simulink model "Boost_model_closed"  (R2021a)
settings: Solver=VariableStepAuto  StartTime=0.0  StopTime=100*1e-3  FixedStep=1e-6  MaxStep=1e-7  RelTol=1e-3
undefined symbols (not defined in the file): bits, DCR, ESR_Cout, f_s, general, gmis_v, K_i_0, K_p_0, nlsb_v, ofs_v, sat_v, T_A2D, t_f, T_PWM, tf1, V_out, V_out_p
libraries: fl_lib x14, ee_lib x8, nesl_utility x6, spsPWMGeneratorDCDCLib x2
settings Model: Creator=delta  LastModifiedBy=delta
settings SolverCC: MaxConsecutiveMinStep=10  ZeroCrossAlgorithm=Adaptive
settings DebuggingCC: IgnoredZcDiagnostic=none  ParameterOverflowMsg=warning

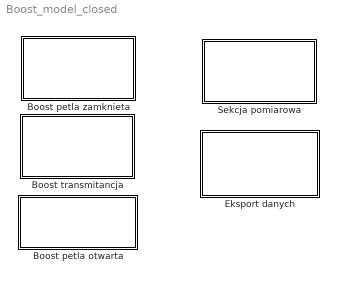
== system Boost_model_closed ==
  Boost petla otwarta : Subsystem
  Boost petla zamknieta : Subsystem
  Boost transmitancja : Subsystem
  Eksport danych : Subsystem
  Sekcja pomiarowa : Subsystem

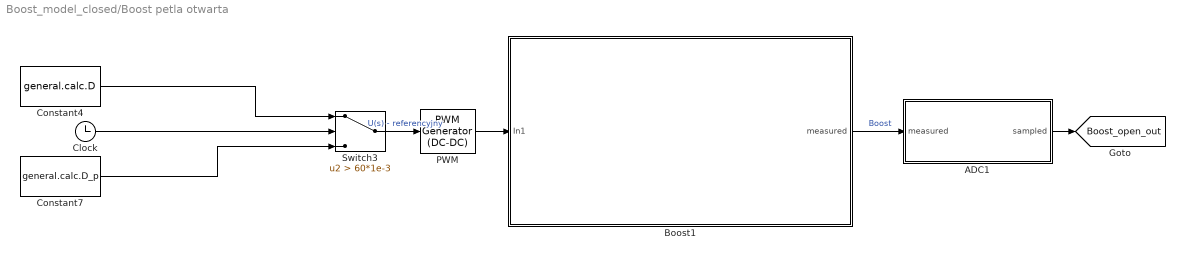
== system Boost_model_closed/Boost petla otwarta ==
  ADC1 : Subsystem
  Boost1 : Subsystem
  Clock : Clock
  Constant4 : Constant  Value=general.calc.D
  Constant7 : Constant  Value=general.calc.D_p
  "PWM " : spsPWMGeneratorDCDCLib/PWM Generator (DC-DC)  Fsw=1/T_PWM  Ts=0
  Switch3 : Switch  Criteria=u2 > Threshold  Threshold=60*1e-3
  tag scope: Boost_open_out=global
  wires:
  ADC1/1(sampled) -> [Boost_open_out]
  Switch3/1 -> "PWM "/1  "U(s) - referencyjny"
  "PWM "/1 -> Boost1/1(In1)
  Clock/1 -> Switch3/2
  Constant4/1 -> Switch3/1
  Boost1/1(measured) -> ADC1/1(measured)  "Boost"
  Constant7/1 -> Switch3/3

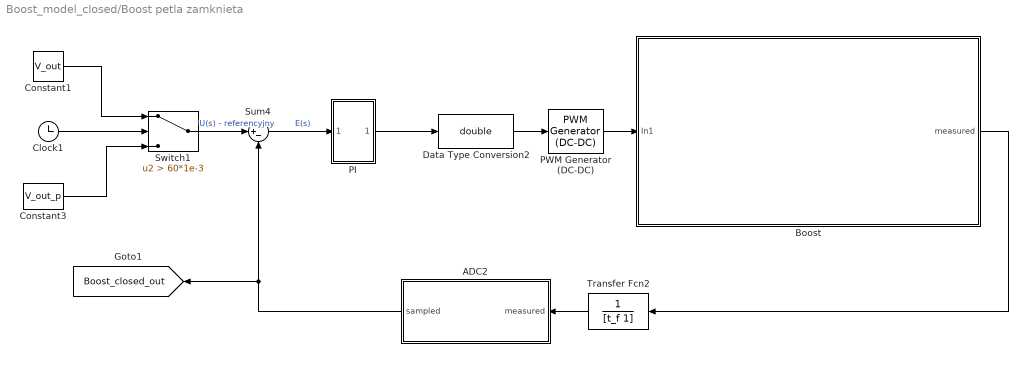
== system Boost_model_closed/Boost petla zamknieta ==
  ADC2 : Subsystem
  Boost : Subsystem
  Clock1 : Clock
  Constant1 : Constant  Value=V_out
  Constant3 : Constant  Value=V_out_p
  Data Type Conversion2 : DataTypeConversion  OutDataTypeStr=double
  PI : Subsystem
  PWM Generator (DC-DC) : spsPWMGeneratorDCDCLib/PWM Generator (DC-DC)  Fsw=1/T_PWM  Ts=0
  Sum4 : Sum  Inputs=|+-
  Switch1 : Switch  Criteria=u2 > Threshold  Threshold=60*1e-3
  Transfer Fcn2 : TransferFcn  Numerator=1  Denominator=[t_f 1]
  tag scope: Boost_closed_out=global
  wires:
  PI/1(Out1) -> Data Type Conversion2/1
  Sum4/1 -> PI/1(In1)  "E(s)"
  Boost/1(measured) -> Transfer Fcn2/1
  Constant3/1 -> Switch1/3
  Clock1/1 -> Switch1/2
  Constant1/1 -> Switch1/1
  ADC2/1(sampled) -> [Boost_closed_out], Sum4/2
  PWM Generator (DC-DC)/1 -> Boost/1(In1)
  Switch1/1 -> Sum4/1  "U(s) - referencyjny"
  Data Type Conversion2/1 -> PWM Generator (DC-DC)/1
  Transfer Fcn2/1 -> ADC2/1(measured)

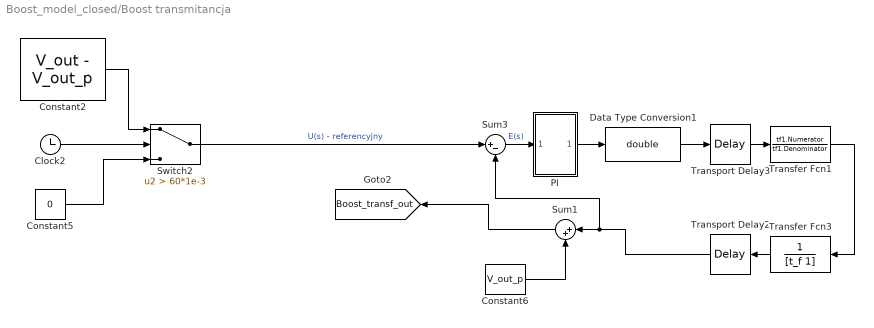
== system Boost_model_closed/Boost transmitancja ==
  Clock2 : Clock
  Constant2 : Constant  Value=V_out - V_out_p
  Constant5 : Constant  Value=0
  Constant6 : Constant  Value=V_out_p
  Data Type Conversion1 : DataTypeConversion  OutDataTypeStr=double
  PI : Subsystem
  Sum1 : Sum  Inputs=|++
  Sum3 : Sum  Inputs=|+-
  Switch2 : Switch  Criteria=u2 > Threshold  Threshold=60*1e-3
  Transfer Fcn1 : TransferFcn  Numerator=tf1.Numerator  Denominator=tf1.Denominator
  Transfer Fcn3 : TransferFcn  Numerator=1  Denominator=[t_f 1]
  Transport Delay2 : TransportDelay  DelayTime=T_A2D
  Transport Delay3 : TransportDelay  DelayTime=T_PWM
  tag scope: Boost_transf_out=global
  wires:
  Transport Delay3/1 -> Transfer Fcn1/1
  PI/1(Out1) -> Data Type Conversion1/1
  Constant5/1 -> Switch2/3
  Switch2/1 -> Sum3/1  "U(s) - referencyjny"
  Constant6/1 -> Sum1/2
  Clock2/1 -> Switch2/2
  Transport Delay2/1 -> Sum3/2, Sum1/1
  Sum3/1 -> PI/1(In1)  "E(s)"
  Transfer Fcn3/1 -> Transport Delay2/1
  Data Type Conversion1/1 -> Transport Delay3/1
  Constant2/1 -> Switch2/1
  Transfer Fcn1/1 -> Transfer Fcn3/1
  Sum1/1 -> [Boost_transf_out]

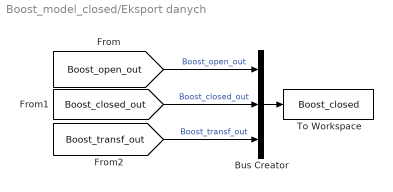
== system Boost_model_closed/Eksport danych ==
  Bus Creator : BusCreator  Inputs=3
  To Workspace : ToWorkspace  VariableName=Boost_closed  SaveFormat=Timeseries  SampleTime=-1
  wires:
  Bus Creator/1 -> To Workspace/1
  [Boost_closed_out] -> Bus Creator/2  "Boost_closed_out"
  [Boost_transf_out] -> Bus Creator/3  "Boost_transf_out"
  [Boost_open_out] -> Bus Creator/1  "Boost_open_out"

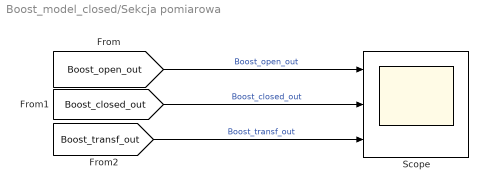
== system Boost_model_closed/Sekcja pomiarowa ==
  Scope : Scope  NumInputPorts=3
  wires:
  [Boost_open_out] -> Scope/1  "Boost_open_out"
  [Boost_transf_out] -> Scope/3  "Boost_transf_out"
  [Boost_closed_out] -> Scope/2  "Boost_closed_out"

== system Boost_model_closed/Boost petla otwarta/ADC1 ==
  measured : Inport
  Discrete Pulse Generator1 : DiscretePulseGenerator  PulseType=Time based  Period=1/f_s  PulseWidth=0.0001
  Triggered Subsystem : Subsystem  TreatAsAtomicUnit=on
  sampled : Outport
  wires:
  Triggered Subsystem/1(sampled) -> sampled/1
  Discrete Pulse Generator1/1 -> Triggered Subsystem/Trigger
  measured/1 -> Triggered Subsystem/1(measured)

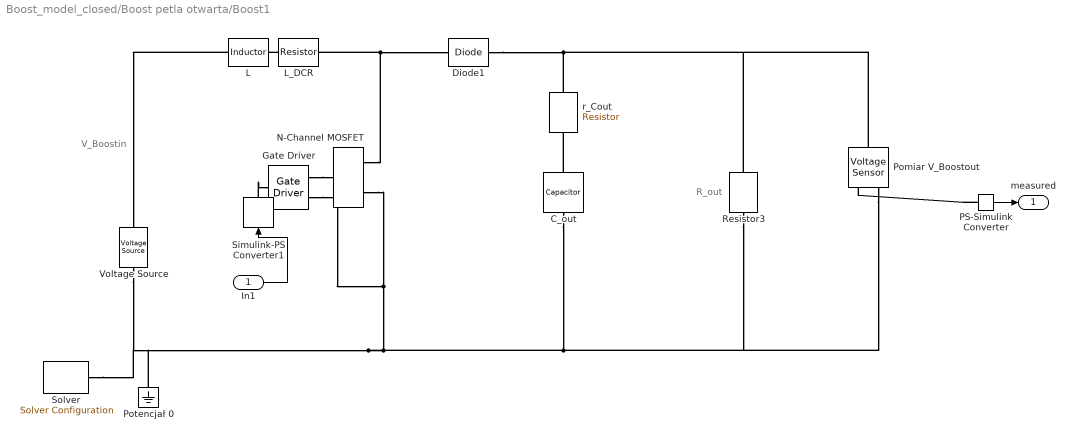
== system Boost_model_closed/Boost petla otwarta/Boost1 ==
  note: V_Boostin
  note: R_out
  In1 : Inport
  "C_out " : fl_lib/Electrical/Electrical Elements/Capacitor  c=C_out F  r=0 Ohm  g=0 1/Ohm  i_specify=off  i_priority=None  i=0 A  i_nominal_specify=off  i_nominal_unit=A  i_nominal_value=1  v_specify=off  v_priority=None  v=0 V  v_nominal_specify=off  v_nominal_unit=V  v_nominal_value=1  vc_specify=off  vc_priority=High  vc=0 V  vc_nominal_specify=off  vc_nominal_unit=V  vc_nominal_value=1
  Diode1 : ee_lib/Semiconductors & Converters/Diode  ModelType=ee.enum.diode.modelType.pwl  IfMat=[.07, .12, .19, 1.75, 4.24, 7.32, 11.2; .16, .3, .72, 2.14, 4.02, 6.35, 9.12] A  TjVec=[25, 125] degC  VfVec=[.5, .7, .9, 1.3, 1.7, 2.1, 2.5] V  Vf=V_f V  Ron=1e-9 Ohm  Goff=1e-8 S  prmExp=ee.enum.diode.expParam.useTwo  I12=[.0137, .545] A  V12=[.6, .7] V  IS=1e-12 A  ec=1  I1=0.0137 A  V1=0.6 V  RS=0 Ohm  Tmeas=25 degC  N_series=1  N_parallel=1  Rz=0.3 Ohm  BV=inf V  C_param=ee.enum.diode.capParam.fixed  CJ=5 pF  CJ0=5 pF  VJ=1 V  Mgrad=0.5  Vvec=[.1, 10, 100] V  Cvec=[3.5, 1, .4] pF  FC=0.5  Q_param=ee.enum.diode.recoveryParam.off  iRM=-7.15 A  iF=4 A  didt=-750 A/us  trr_factor=3  trr=115 ns  Qrr=150 s*nA  TT=50 ns  tau=100 ns  T_param=ee.enum.diode.temperatureParam.off  IS_T2=1.25e-7 A  I1_T2=0.245 A  V1_T2=0.5 V  Tmeas2=125 degC  EG_param=ee.enum.diode.egapParam.material_si  EG=1.11 eV  XTI_param=ee.enum.diode.xtiParam.pn  XTI=3  dBVdT=0 V/K  enable_faults=ee.enum.faults.faultEnable.no  fault_action=ee.enum.faults.faultAction.none  fault_types=ee.enum.diode.faults.open  tau_fault=1e-3 s  IfMat_faulted=[.07, .12, .19, 1.75, 4.24, 7.32, 11.2; .16, .3, .72, 2.14, 4.02, 6.35, 9.12] A  VfVec_faulted=[.5, .7, .9, 1.3, 1.7, 2.1, 2.5] V  Ropen_faulted=1000 Ohm  Gshort_faulted=1000 1/Ohm  Vf_faulted=0.6 V  Ron_faulted=0.3 Ohm  Goff_faulted=1e-8 S  I12_faulted=[.0137, .545] A  V12_faulted=[.6, .7] V  IS_faulted=1e-12 A  ec_faulted=1  I1_faulted=0.0137 A  V1_faulted=0.6 V  RS_faulted=0 Ohm  Rz_faulted=0.3 Ohm  BV_faulted=inf V  Cscale_faulted=100  enable_temporal_fault=ee.enum.faults.faultEnable.no  t_fault=inf s  enable_behavioral_fault=ee.enum.faults.faultEnable.no  max_permissible_voltage=inf V  n_fail_on_voltage=1  max_permissible_current=inf A  t_fail_on_current=1 s  max_permissible_dVdt=inf V/s  Tdevice=25 degC  i_specify=off  i_priority=None  i=0 A  i_nominal_specify=off  i_nominal_unit=A  i_nominal_value=1  v_specify=off  v_priority=None  v=0 V  v_nominal_specify=off  v_nominal_unit=V  v_nominal_value=1  i_diode_specify=off  i_diode_priority=None  i_diode=0 A  i_diode_nominal_specify=off  i_diode_nominal_unit=A  i_diode_nominal_value=1  v_diode_specify=off  v_diode_priority=None  v_diode=0 V  v_diode_nominal_specify=off  v_diode_nominal_unit=V  v_diode_nominal_value=1  i_capacitor_specify=off  i_capacitor_priority=None  i_capacitor=0 A  i_capacitor_nominal_specify=off  i_capacitor_nominal_unit=A  i_capacitor_nominal_value=1  v_capacitor_specify=off  v_capacitor_priority=None  v_capacitor=0 V  v_capacitor_nominal_specify=off  v_capacitor_nominal_unit=V  v_capacitor_nominal_value=1  power_dissipated_specify=off  power_dissipated_priority=None  power_dissipated=0 W  power_dissipated_nominal_specify=off  power_dissipated_nominal_unit=W  power_dissipated_nominal_value=1  max_permissible_temperature=inf K  t_fail_on_temperature=1 s  thermal_network_parameterization=ee.enum.thermalNetworkTopology.cauer  Rth=[0, 10] K/W  Rth_Foster=[4, 6] K/W  thermal_mass_parameterization=ee.enum.thermalNetwork.timeconstant  thermal_mass=[0, 1] J/K  thermal_mass_Foster=[1.5, 3] J/K  thermal_time_constant=[0, 10] s  thermal_time_constant_Foster=[6, 18] s  thermal_mass_initial_temperatures=[25, 25] degC
  Gate Driver : ee_lib/Semiconductors & Converters/Gate Driver  vHigh=V_GS V  vLow=0 V  parameterization=2  rHigh=1e-9 Ohm  rLow=1e-9 Ohm  tRise=t_R s  tFall=t_F s  cLoad=10 nF  enable_faults=0  t_fault=1 s  fault_type=1  uHighValue=0.7  uLowValue=0.3  tHigh=t_R s  tLow=t_F s  ZonTime_specify=off  ZonTime_priority=None  ZonTime=0 s  ZoffTime_specify=off  ZoffTime_priority=None  ZoffTime=0 s  uHigh=2.0 V  uLow=0.8 V
      settings: SourceProductBaseCode=PS  InternalSimscapePortConfiguration="{\"Bottom\":[],\"Left\":[{\"id\":\"u\",\"label\":\"u\",\"type\":\"input\"}],\"Right\":[{\"id\":\"G\",\"label\":\"G\",\"type\":\"foundation.electrical.electrical\"},{\"id\":\"S\",\"label\":\"S\",\"type\":\"foundation.electrical.electrical\"}],\"Top\":[]}"
  L : fl_lib/Electrical/Electrical Elements/Inductor  l=L.param.L H  r=0 Ohm  g=0 1/Ohm  i_specify=off  i_priority=None  i=0 A  i_nominal_specify=off  i_nominal_unit=A  i_nominal_value=1  v_specify=off  v_priority=None  v=0 V  v_nominal_specify=off  v_nominal_unit=V  v_nominal_value=1  i_L_specify=off  i_L_priority=High  i_L=0 A  i_L_nominal_specify=off  i_L_nominal_unit=A  i_L_nominal_value=1
  L_DCR : fl_lib/Electrical/Electrical Elements/Resistor  R=DCR Ohm  i_specify=off  i_priority=None  i=0 A  i_nominal_specify=off  i_nominal_unit=A  i_nominal_value=1  v_specify=off  v_priority=None  v=0 V  v_nominal_specify=off  v_nominal_unit=V  v_nominal_value=1
  N-Channel MOSFET : ee_lib/Semiconductors & Converters/N-Channel MOSFET  paramTerminal=ee.enum.mosfet.numberOfTerminals.three  parameterization=ee.enum.mosfet.parameterization.datasheet  prmDatasheet=ee.enum.temperatureParameterization.none  prmEquCoeff=ee.enum.temperatureParameterization.none  Beta=5.0 A/V^2  Rds=R_DS Ohm  Id=I_D A  Vgs=V_GS V  Vth=V_th V  Vth0=1.7 V  lam=0 1/V  gamma_vth=0.5 V^0.50000  phib=0.5 V  Vth1=1.9071 V  Vbs1=-1 V  Vth2=2.066 V  Vbs2=-2 V  Tmeas=25 degC  RS=1e-9 Ohm  RD=1e-9 Ohm  RB=0.001 Ohm  C_param=ee.enum.mosfet.capacitanceParam.fixedciss  C_GS=270 pF  C_GD=80 pF  C_DS=0 pF  C_iss=C_iss F  C_rss=C_rss F  C_oss=C_oss F  charge_linearity_param=ee.enum.mosfet.cgdLinearity.constant  C_OX=200 pF  V_C_OX=-0.5 V  C_iss_vec=[720, 700, 590, 470, 390, 310] pF  C_rss_vec=[450, 400, 300, 190, 95, 55] pF  C_oss_vec=[900, 810, 690, 420, 270, 170] pF  C_GS_vec=[270, 300, 290, 280, 295, 255] pF  C_GD_vec=[450, 400, 300, 190, 95, 55] pF  C_DS_vec=[450, 410, 390, 230, 175, 115] pF  C_Vds_vec=[.1, .3, 1, 3, 10, 30] V  V_GS_for_cap_data=0 V  charge_linearity_param_vgb=ee.enum.mosfet.cgbLinearity.instantly  Di_param=ee.enum.mosfet.diodeParam.no  IsDiode=0 A  Vbi=0.6 V  n=1  Cj0Diode=0 pF  TT=50e-9 s  dVth_dT=-6 mV/K  dVth0_dT=-6 mV/K  Rds_T2=0.037 Ohm  Tmeas2=125 degC  BEXDatasheet=-1.5  BEXEquCoeff=-1.5  etaisDatasheet=3  etaisEquCoeff=3  Vgs_vec=[-.5, 2, 3, 4, 5] V  Vds_vec=[0, 2, 4, 8, 12, 16, 20] V  Vbs_vec=[0, -4, -6, -12] V  T_vec=[25, 125] degC  Vth_vec=[.4, 1.2, 1.4, 1.45] V  Vth_mat=[.4, .35; 1.2, 1.15; 1.4, 1.35; 1.45, 1.4] V  Ids_mat=[0, 0, 0, 0, 0, 0, 0; 0, .003, .0038, .0043, .0046, .0048, .0049; 0, .0055, .008, .009, .0095, .01, .0101; 0, .0115, .016, .018, .019, .0195, .02; 0, .0152, .0225, .0265, .028, .0295, .03] A  Ids_mat0=[0, 0, 0, 0, 0, 0, 0; 0, .003, .0038, .0043, .0046, .0048, .0049; 0, .0055, .008, .009, .0095, .01, .0101; 0, .0115, .016, .018, .019, .0195, .02; 0, .0152, .0225, .0265, .028, .0295, .03] A  Ids_mat_3D=zeros(5, 7, 2) A  Ids_mat_3D0=zeros(5, 7, 2) A  IV_table_symmetry=ee.enum.mosfet.symmetricNIV.no  VfVec=[.5, .7, .9, 1.3, 1.7, 2.1, 2.5] V  TjVec=[25, 125] degC  IfVec=[.07, .12, .19, 1.75, 4.24, 7.32, 11.2] A  IfMat=[.07, .12, .19, 1.75, 4.24, 7.32, 11.2; .16, .3, .72, 2.14, 4.02, 6.35, 9.12] A  Tmeas_dio=25 degC  etaisTabulated=3  TdeviceDatasheet=25 degC  TdeviceEquCoeff=25 degC  TdeviceTabulated=25 degC  thermal_network_parameterization=ee.enum.thermalNetworkTopology.cauer  Rth=[0, 10] K/W  Rth_Foster=[4, 6] K/W  thermal_mass_parameterization=ee.enum.thermalNetwork.timeconstant  thermal_mass=[0, 1] J/K  thermal_mass_Foster=[1.5, 3] J/K  thermal_time_constant=[0, 10] s  thermal_time_constant_Foster=[6, 18] s  thermal_mass_initial_temperatures=[25, 25] degC  betaref=18 A/V^2  Vfbref=-1.1 V  gamma=3.5 V^0.50000  phib2ref=1 V  thesatref=0.4 1/V  alpha=0  Vp=5e-2 V  thesrref=0 1/V  m=8  Tref=25 degC  Cox=1500 pF  Cgso=100 pF  Cgdo=14 pF  Rsref=2e-3 Ohm  Rdref=0.17 Ohm  Rgref=8.4 Ohm  Rbref=2e-3 Ohm  Isref=5.2e-13 A  Cj0=480 pF  Tprm=1  etabet=1.3  Stvfb=5e-4 V/K  Stphib=-8.5e-4 V/K  etasat=1.04  etasr=0.65  etar=0.95  etais=3  Tsim=25 degC  T0=[25, 25] degC
  PS-Simulink Converter : nesl_utility/PS-Simulink Converter  PhysicalDomain=network_engine_domain  SubClassName=ps_output  LeftPortType=input  RightPortType=output  PseudoPeriodic=off  Frequencies=[]  Unit=inherit  AffineConversion=off
      settings: SourceProductBaseCode=PW,SS
  "Pomiar V_Boostout " : fl_lib/Electrical/Electrical Sensors/Voltage Sensor
  Potencjał 0 : fl_lib/Electrical/Electrical Elements/Electrical Reference
  Resistor3 : fl_lib/Electrical/Electrical Elements/Resistor  R=22.5 Ohm  i_specify=off  i_priority=None  i=0 A  i_nominal_specify=off  i_nominal_unit=A  i_nominal_value=1  v_specify=off  v_priority=None  v=0 V  v_nominal_specify=off  v_nominal_unit=V  v_nominal_value=1
  Simulink-PS Converter1 : nesl_utility/Simulink-PS Converter  PhysicalDomain=network_engine_domain  SubClassName=ps_input  LeftPortType=input  RightPortType=output  PseudoPeriodic=off  Frequencies=[]  NoiseDistribution=none  NoiseParameters=[]  Unit=1  AffineConversion=off  FilteringAndDerivatives=provide  SimscapeFilterOrder=1  InputFilterTimeConstant=0.001  UdotUserProvided=0
  "Solver " : nesl_utility/Solver Configuration  PhysicalDomain=network_engine_domain  SubClassName=solver  LeftPortType=input  RightPortType=generic  Tones=[]  Harmonics=[]  SimulateNoise=off  Profile=off  UseLocalSampling=off  EnableSwitchedLinearOptims=on  FrequencyDomain=off  UseCCode=off  RelTol=0.001  AbsTol=1e-06  MinStep=1e-09  ToWorkspace=off  RevertToSquareIcSolve=off  NumHomotopyIterations=100  PhasorMode=off  PhasorModeNumHarmonics=1  DoDC=off  ResidualTolerance=1e-09  UseLocalSolver=off  LocalSolverChoice=NE_BACKWARD_EULER_ADVANCER  LocalSolverSampleTime=0.001  DoFixedCost=on  MaxNonlinIter=3  MaxModeIter=2  ComputeImpulses=off  ImpulseIterations=2  LinearAlgebra=auto  EquationFormulation=NE_TIME_EF  DelaysMemoryBudget=1024  AutomaticFiltering=on  FilteringTimeConstant=0.001  PartitionStorageMethod=AS_NEEDED  PartitionMemoryBudget=1024  PartitionMethod=ROBUST
      settings: SourceProductBaseCode=PW,SS
  Voltage Source : ee_lib/Sources/Voltage Source  dc_voltage=30 V  ac_voltage=0 V  ac_shift=0 rad  ac_frequency=60 Hz  noise_mode=0  PSD=0.2/1e3 V^2/Hz  repeatability=1  auto_seed=2032760128  user_seed=0  sample_time=1e-3 s  i_specify=off  i_priority=None  i=0 A  i_nominal_specify=off  i_nominal_unit=A  i_nominal_value=1  v_specify=off  v_priority=None  v=0 V  v_nominal_specify=off  v_nominal_unit=V  v_nominal_value=1
  r_Cout : fl_lib/Electrical/Electrical Elements/Resistor  R=ESR_Cout Ohm  i_specify=off  i_priority=None  i=0 A  i_nominal_specify=off  i_nominal_unit=A  i_nominal_value=1  v_specify=off  v_priority=None  v=0 V  v_nominal_specify=off  v_nominal_unit=V  v_nominal_value=1
  measured : Outport
  wires:
  PS-Simulink Converter/1 -> measured/1
  In1/1 -> Simulink-PS Converter1/1
  connections:
  N-Channel MOSFET/RConn2 -- Gate Driver/RConn2 -- "Solver "/RConn1 -- Voltage Source/RConn1 -- Potencjał 0/LConn1 -- Resistor3/RConn1 -- "Pomiar V_Boostout "/RConn2 -- "C_out "/RConn1
  "C_out "/LConn1 -- r_Cout/RConn1
  PS-Simulink Converter/LConn1 -- "Pomiar V_Boostout "/RConn1
  Diode1/RConn1 -- r_Cout/LConn1 -- Resistor3/LConn1 -- "Pomiar V_Boostout "/LConn1
  L_DCR/LConn1 -- L/RConn1
  N-Channel MOSFET/RConn1 -- L_DCR/RConn1 -- Diode1/LConn1
  L/LConn1 -- Voltage Source/LConn1
  Simulink-PS Converter1/RConn1 -- Gate Driver/LConn1
  Gate Driver/RConn1 -- N-Channel MOSFET/LConn1

== system Boost_model_closed/Boost petla zamknieta/ADC2 ==
  measured : Inport
  Discrete Pulse Generator1 : DiscretePulseGenerator  PulseType=Time based  Period=1/f_s  PulseWidth=0.0001
  Triggered Subsystem : Subsystem  TreatAsAtomicUnit=on
  sampled : Outport
  wires:
  Triggered Subsystem/1(sampled) -> sampled/1
  Discrete Pulse Generator1/1 -> Triggered Subsystem/Trigger
  measured/1 -> Triggered Subsystem/1(measured)

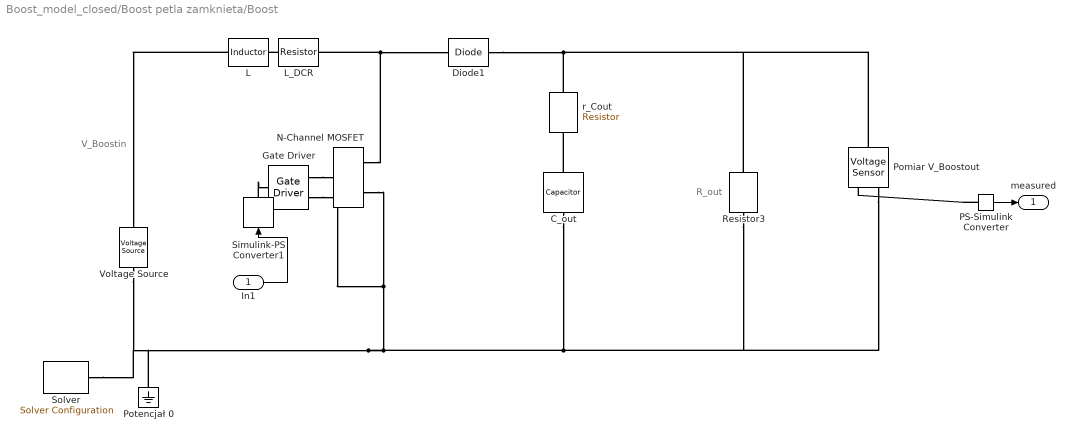
== system Boost_model_closed/Boost petla zamknieta/Boost ==
  note: V_Boostin
  note: R_out
  In1 : Inport
  "C_out " : fl_lib/Electrical/Electrical Elements/Capacitor  c=C_out F  r=0 Ohm  g=0 1/Ohm  i_specify=off  i_priority=None  i=0 A  i_nominal_specify=off  i_nominal_unit=A  i_nominal_value=1  v_specify=off  v_priority=None  v=0 V  v_nominal_specify=off  v_nominal_unit=V  v_nominal_value=1  vc_specify=off  vc_priority=High  vc=0 V  vc_nominal_specify=off  vc_nominal_unit=V  vc_nominal_value=1
  Diode1 : ee_lib/Semiconductors & Converters/Diode  ModelType=ee.enum.diode.modelType.pwl  IfMat=[.07, .12, .19, 1.75, 4.24, 7.32, 11.2; .16, .3, .72, 2.14, 4.02, 6.35, 9.12] A  TjVec=[25, 125] degC  VfVec=[.5, .7, .9, 1.3, 1.7, 2.1, 2.5] V  Vf=V_f V  Ron=1e-9 Ohm  Goff=1e-8 S  prmExp=ee.enum.diode.expParam.useTwo  I12=[.0137, .545] A  V12=[.6, .7] V  IS=1e-12 A  ec=1  I1=0.0137 A  V1=0.6 V  RS=0 Ohm  Tmeas=25 degC  N_series=1  N_parallel=1  Rz=0.3 Ohm  BV=inf V  C_param=ee.enum.diode.capParam.fixed  CJ=5 pF  CJ0=5 pF  VJ=1 V  Mgrad=0.5  Vvec=[.1, 10, 100] V  Cvec=[3.5, 1, .4] pF  FC=0.5  Q_param=ee.enum.diode.recoveryParam.off  iRM=-7.15 A  iF=4 A  didt=-750 A/us  trr_factor=3  trr=115 ns  Qrr=150 s*nA  TT=50 ns  tau=100 ns  T_param=ee.enum.diode.temperatureParam.off  IS_T2=1.25e-7 A  I1_T2=0.245 A  V1_T2=0.5 V  Tmeas2=125 degC  EG_param=ee.enum.diode.egapParam.material_si  EG=1.11 eV  XTI_param=ee.enum.diode.xtiParam.pn  XTI=3  dBVdT=0 V/K  enable_faults=ee.enum.faults.faultEnable.no  fault_action=ee.enum.faults.faultAction.none  fault_types=ee.enum.diode.faults.open  tau_fault=1e-3 s  IfMat_faulted=[.07, .12, .19, 1.75, 4.24, 7.32, 11.2; .16, .3, .72, 2.14, 4.02, 6.35, 9.12] A  VfVec_faulted=[.5, .7, .9, 1.3, 1.7, 2.1, 2.5] V  Ropen_faulted=1000 Ohm  Gshort_faulted=1000 1/Ohm  Vf_faulted=0.6 V  Ron_faulted=0.3 Ohm  Goff_faulted=1e-8 S  I12_faulted=[.0137, .545] A  V12_faulted=[.6, .7] V  IS_faulted=1e-12 A  ec_faulted=1  I1_faulted=0.0137 A  V1_faulted=0.6 V  RS_faulted=0 Ohm  Rz_faulted=0.3 Ohm  BV_faulted=inf V  Cscale_faulted=100  enable_temporal_fault=ee.enum.faults.faultEnable.no  t_fault=inf s  enable_behavioral_fault=ee.enum.faults.faultEnable.no  max_permissible_voltage=inf V  n_fail_on_voltage=1  max_permissible_current=inf A  t_fail_on_current=1 s  max_permissible_dVdt=inf V/s  Tdevice=25 degC  i_specify=off  i_priority=None  i=0 A  i_nominal_specify=off  i_nominal_unit=A  i_nominal_value=1  v_specify=off  v_priority=None  v=0 V  v_nominal_specify=off  v_nominal_unit=V  v_nominal_value=1  i_diode_specify=off  i_diode_priority=None  i_diode=0 A  i_diode_nominal_specify=off  i_diode_nominal_unit=A  i_diode_nominal_value=1  v_diode_specify=off  v_diode_priority=None  v_diode=0 V  v_diode_nominal_specify=off  v_diode_nominal_unit=V  v_diode_nominal_value=1  i_capacitor_specify=off  i_capacitor_priority=None  i_capacitor=0 A  i_capacitor_nominal_specify=off  i_capacitor_nominal_unit=A  i_capacitor_nominal_value=1  v_capacitor_specify=off  v_capacitor_priority=None  v_capacitor=0 V  v_capacitor_nominal_specify=off  v_capacitor_nominal_unit=V  v_capacitor_nominal_value=1  power_dissipated_specify=off  power_dissipated_priority=None  power_dissipated=0 W  power_dissipated_nominal_specify=off  power_dissipated_nominal_unit=W  power_dissipated_nominal_value=1  max_permissible_temperature=inf K  t_fail_on_temperature=1 s  thermal_network_parameterization=ee.enum.thermalNetworkTopology.cauer  Rth=[0, 10] K/W  Rth_Foster=[4, 6] K/W  thermal_mass_parameterization=ee.enum.thermalNetwork.timeconstant  thermal_mass=[0, 1] J/K  thermal_mass_Foster=[1.5, 3] J/K  thermal_time_constant=[0, 10] s  thermal_time_constant_Foster=[6, 18] s  thermal_mass_initial_temperatures=[25, 25] degC
  Gate Driver : ee_lib/Semiconductors & Converters/Gate Driver  vHigh=V_GS V  vLow=0 V  parameterization=2  rHigh=1e-9 Ohm  rLow=1e-9 Ohm  tRise=t_R s  tFall=t_F s  cLoad=10 nF  enable_faults=0  t_fault=1 s  fault_type=1  uHighValue=0.7  uLowValue=0.3  tHigh=t_R s  tLow=t_F s  ZonTime_specify=off  ZonTime_priority=None  ZonTime=0 s  ZoffTime_specify=off  ZoffTime_priority=None  ZoffTime=0 s  uHigh=2.0 V  uLow=0.8 V
      settings: SourceProductBaseCode=PS  InternalSimscapePortConfiguration="{\"Bottom\":[],\"Left\":[{\"id\":\"u\",\"label\":\"u\",\"type\":\"input\"}],\"Right\":[{\"id\":\"G\",\"label\":\"G\",\"type\":\"foundation.electrical.electrical\"},{\"id\":\"S\",\"label\":\"S\",\"type\":\"foundation.electrical.electrical\"}],\"Top\":[]}"
  L : fl_lib/Electrical/Electrical Elements/Inductor  l=L.param.L H  r=0 Ohm  g=0 1/Ohm  i_specify=off  i_priority=None  i=0 A  i_nominal_specify=off  i_nominal_unit=A  i_nominal_value=1  v_specify=off  v_priority=None  v=0 V  v_nominal_specify=off  v_nominal_unit=V  v_nominal_value=1  i_L_specify=off  i_L_priority=High  i_L=0 A  i_L_nominal_specify=off  i_L_nominal_unit=A  i_L_nominal_value=1
  L_DCR : fl_lib/Electrical/Electrical Elements/Resistor  R=DCR Ohm  i_specify=off  i_priority=None  i=0 A  i_nominal_specify=off  i_nominal_unit=A  i_nominal_value=1  v_specify=off  v_priority=None  v=0 V  v_nominal_specify=off  v_nominal_unit=V  v_nominal_value=1
  N-Channel MOSFET : ee_lib/Semiconductors & Converters/N-Channel MOSFET  paramTerminal=ee.enum.mosfet.numberOfTerminals.three  parameterization=ee.enum.mosfet.parameterization.datasheet  prmDatasheet=ee.enum.temperatureParameterization.none  prmEquCoeff=ee.enum.temperatureParameterization.none  Beta=5.0 A/V^2  Rds=R_DS Ohm  Id=I_D A  Vgs=V_GS V  Vth=V_th V  Vth0=1.7 V  lam=0 1/V  gamma_vth=0.5 V^0.50000  phib=0.5 V  Vth1=1.9071 V  Vbs1=-1 V  Vth2=2.066 V  Vbs2=-2 V  Tmeas=25 degC  RS=1e-9 Ohm  RD=1e-9 Ohm  RB=0.001 Ohm  C_param=ee.enum.mosfet.capacitanceParam.fixedciss  C_GS=270 pF  C_GD=80 pF  C_DS=0 pF  C_iss=C_iss F  C_rss=C_rss F  C_oss=C_oss F  charge_linearity_param=ee.enum.mosfet.cgdLinearity.constant  C_OX=200 pF  V_C_OX=-0.5 V  C_iss_vec=[720, 700, 590, 470, 390, 310] pF  C_rss_vec=[450, 400, 300, 190, 95, 55] pF  C_oss_vec=[900, 810, 690, 420, 270, 170] pF  C_GS_vec=[270, 300, 290, 280, 295, 255] pF  C_GD_vec=[450, 400, 300, 190, 95, 55] pF  C_DS_vec=[450, 410, 390, 230, 175, 115] pF  C_Vds_vec=[.1, .3, 1, 3, 10, 30] V  V_GS_for_cap_data=0 V  charge_linearity_param_vgb=ee.enum.mosfet.cgbLinearity.instantly  Di_param=ee.enum.mosfet.diodeParam.no  IsDiode=0 A  Vbi=0.6 V  n=1  Cj0Diode=0 pF  TT=50e-9 s  dVth_dT=-6 mV/K  dVth0_dT=-6 mV/K  Rds_T2=0.037 Ohm  Tmeas2=125 degC  BEXDatasheet=-1.5  BEXEquCoeff=-1.5  etaisDatasheet=3  etaisEquCoeff=3  Vgs_vec=[-.5, 2, 3, 4, 5] V  Vds_vec=[0, 2, 4, 8, 12, 16, 20] V  Vbs_vec=[0, -4, -6, -12] V  T_vec=[25, 125] degC  Vth_vec=[.4, 1.2, 1.4, 1.45] V  Vth_mat=[.4, .35; 1.2, 1.15; 1.4, 1.35; 1.45, 1.4] V  Ids_mat=[0, 0, 0, 0, 0, 0, 0; 0, .003, .0038, .0043, .0046, .0048, .0049; 0, .0055, .008, .009, .0095, .01, .0101; 0, .0115, .016, .018, .019, .0195, .02; 0, .0152, .0225, .0265, .028, .0295, .03] A  Ids_mat0=[0, 0, 0, 0, 0, 0, 0; 0, .003, .0038, .0043, .0046, .0048, .0049; 0, .0055, .008, .009, .0095, .01, .0101; 0, .0115, .016, .018, .019, .0195, .02; 0, .0152, .0225, .0265, .028, .0295, .03] A  Ids_mat_3D=zeros(5, 7, 2) A  Ids_mat_3D0=zeros(5, 7, 2) A  IV_table_symmetry=ee.enum.mosfet.symmetricNIV.no  VfVec=[.5, .7, .9, 1.3, 1.7, 2.1, 2.5] V  TjVec=[25, 125] degC  IfVec=[.07, .12, .19, 1.75, 4.24, 7.32, 11.2] A  IfMat=[.07, .12, .19, 1.75, 4.24, 7.32, 11.2; .16, .3, .72, 2.14, 4.02, 6.35, 9.12] A  Tmeas_dio=25 degC  etaisTabulated=3  TdeviceDatasheet=25 degC  TdeviceEquCoeff=25 degC  TdeviceTabulated=25 degC  thermal_network_parameterization=ee.enum.thermalNetworkTopology.cauer  Rth=[0, 10] K/W  Rth_Foster=[4, 6] K/W  thermal_mass_parameterization=ee.enum.thermalNetwork.timeconstant  thermal_mass=[0, 1] J/K  thermal_mass_Foster=[1.5, 3] J/K  thermal_time_constant=[0, 10] s  thermal_time_constant_Foster=[6, 18] s  thermal_mass_initial_temperatures=[25, 25] degC  betaref=18 A/V^2  Vfbref=-1.1 V  gamma=3.5 V^0.50000  phib2ref=1 V  thesatref=0.4 1/V  alpha=0  Vp=5e-2 V  thesrref=0 1/V  m=8  Tref=25 degC  Cox=1500 pF  Cgso=100 pF  Cgdo=14 pF  Rsref=2e-3 Ohm  Rdref=0.17 Ohm  Rgref=8.4 Ohm  Rbref=2e-3 Ohm  Isref=5.2e-13 A  Cj0=480 pF  Tprm=1  etabet=1.3  Stvfb=5e-4 V/K  Stphib=-8.5e-4 V/K  etasat=1.04  etasr=0.65  etar=0.95  etais=3  Tsim=25 degC  T0=[25, 25] degC
  PS-Simulink Converter : nesl_utility/PS-Simulink Converter  PhysicalDomain=network_engine_domain  SubClassName=ps_output  LeftPortType=input  RightPortType=output  PseudoPeriodic=off  Frequencies=[]  Unit=inherit  AffineConversion=off
      settings: SourceProductBaseCode=PW,SS
  "Pomiar V_Boostout " : fl_lib/Electrical/Electrical Sensors/Voltage Sensor
  Potencjał 0 : fl_lib/Electrical/Electrical Elements/Electrical Reference
  Resistor3 : fl_lib/Electrical/Electrical Elements/Resistor  R=general.calc.R_out Ohm  i_specify=off  i_priority=None  i=0 A  i_nominal_specify=off  i_nominal_unit=A  i_nominal_value=1  v_specify=off  v_priority=None  v=0 V  v_nominal_specify=off  v_nominal_unit=V  v_nominal_value=1
  Simulink-PS Converter1 : nesl_utility/Simulink-PS Converter  PhysicalDomain=network_engine_domain  SubClassName=ps_input  LeftPortType=input  RightPortType=output  PseudoPeriodic=off  Frequencies=[]  NoiseDistribution=none  NoiseParameters=[]  Unit=1  AffineConversion=off  FilteringAndDerivatives=provide  SimscapeFilterOrder=1  InputFilterTimeConstant=0.001  UdotUserProvided=0
  "Solver " : nesl_utility/Solver Configuration  PhysicalDomain=network_engine_domain  SubClassName=solver  LeftPortType=input  RightPortType=generic  Tones=[]  Harmonics=[]  SimulateNoise=off  Profile=off  UseLocalSampling=off  EnableSwitchedLinearOptims=on  FrequencyDomain=off  UseCCode=off  RelTol=0.001  AbsTol=1e-06  MinStep=1e-09  ToWorkspace=off  RevertToSquareIcSolve=off  NumHomotopyIterations=100  PhasorMode=off  PhasorModeNumHarmonics=1  DoDC=off  ResidualTolerance=1e-09  UseLocalSolver=off  LocalSolverChoice=NE_BACKWARD_EULER_ADVANCER  LocalSolverSampleTime=0.001  DoFixedCost=on  MaxNonlinIter=3  MaxModeIter=2  ComputeImpulses=off  ImpulseIterations=2  LinearAlgebra=auto  EquationFormulation=NE_TIME_EF  DelaysMemoryBudget=1024  AutomaticFiltering=on  FilteringTimeConstant=0.001  PartitionStorageMethod=AS_NEEDED  PartitionMemoryBudget=1024  PartitionMethod=ROBUST
      settings: SourceProductBaseCode=PW,SS
  Voltage Source : ee_lib/Sources/Voltage Source  dc_voltage=30 V  ac_voltage=0 V  ac_shift=0 rad  ac_frequency=60 Hz  noise_mode=0  PSD=0.2/1e3 V^2/Hz  repeatability=1  auto_seed=2816384857  user_seed=0  sample_time=1e-3 s  i_specify=off  i_priority=None  i=0 A  i_nominal_specify=off  i_nominal_unit=A  i_nominal_value=1  v_specify=off  v_priority=None  v=0 V  v_nominal_specify=off  v_nominal_unit=V  v_nominal_value=1
  r_Cout : fl_lib/Electrical/Electrical Elements/Resistor  R=ESR_Cout Ohm  i_specify=off  i_priority=None  i=0 A  i_nominal_specify=off  i_nominal_unit=A  i_nominal_value=1  v_specify=off  v_priority=None  v=0 V  v_nominal_specify=off  v_nominal_unit=V  v_nominal_value=1
  measured : Outport
  wires:
  PS-Simulink Converter/1 -> measured/1
  In1/1 -> Simulink-PS Converter1/1
  connections:
  N-Channel MOSFET/RConn2 -- Gate Driver/RConn2 -- "Solver "/RConn1 -- Voltage Source/RConn1 -- Potencjał 0/LConn1 -- Resistor3/RConn1 -- "Pomiar V_Boostout "/RConn2 -- "C_out "/RConn1
  "C_out "/LConn1 -- r_Cout/RConn1
  PS-Simulink Converter/LConn1 -- "Pomiar V_Boostout "/RConn1
  Diode1/RConn1 -- r_Cout/LConn1 -- Resistor3/LConn1 -- "Pomiar V_Boostout "/LConn1
  L_DCR/LConn1 -- L/RConn1
  N-Channel MOSFET/RConn1 -- L_DCR/RConn1 -- Diode1/LConn1
  L/LConn1 -- Voltage Source/LConn1
  Simulink-PS Converter1/RConn1 -- Gate Driver/LConn1
  Gate Driver/RConn1 -- N-Channel MOSFET/LConn1

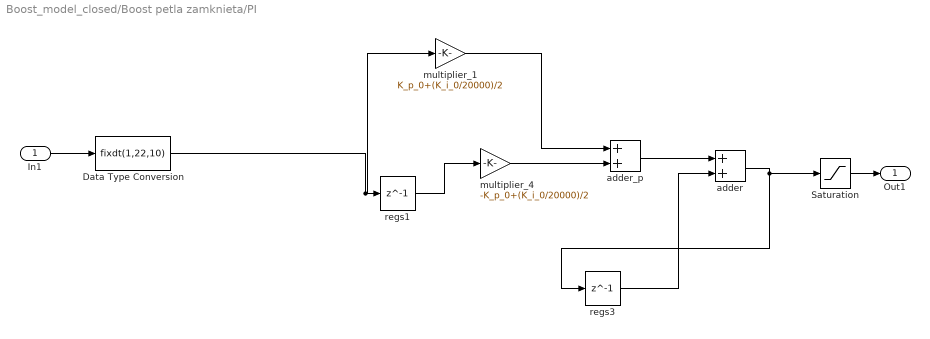
== system Boost_model_closed/Boost petla zamknieta/PI ==
  In1 : Inport
  Data Type Conversion : DataTypeConversion  OutDataTypeStr=fixdt(1,22,10)
  Saturation : Saturate  UpperLimit=1  LowerLimit=0
  adder : Sum  AccumDataTypeStr=fixdt(1,42,30)  OutDataTypeStr=fixdt(1,42,30)
  adder_p : Sum  AccumDataTypeStr=fixdt(1,42,30)  OutDataTypeStr=fixdt(1,42,30)
  multiplier_1 : Gain  Gain=K_p_0+(K_i_0/20000)/2  ParamDataTypeStr=fixdt(1,21,20)  OutDataTypeStr=fixdt(1,42,30)
  multiplier_4 : Gain  Gain=-K_p_0+(K_i_0/20000)/2  ParamDataTypeStr=fixdt(1,21,20)  OutDataTypeStr=fixdt(1,42,30)
  regs1 : Delay  DelayLength=1  SampleTime=T_PWM
  regs3 : Delay  DelayLength=1  SampleTime=T_PWM
  Out1 : Outport
  wires:
  multiplier_1/1 -> adder_p/1
  multiplier_4/1 -> adder_p/2
  adder/1 -> Saturation/1, regs3/1
  adder_p/1 -> adder/1
  Data Type Conversion/1 -> multiplier_1/1, regs1/1
  regs1/1 -> multiplier_4/1
  regs3/1 -> adder/2
  Saturation/1 -> Out1/1
  In1/1 -> Data Type Conversion/1

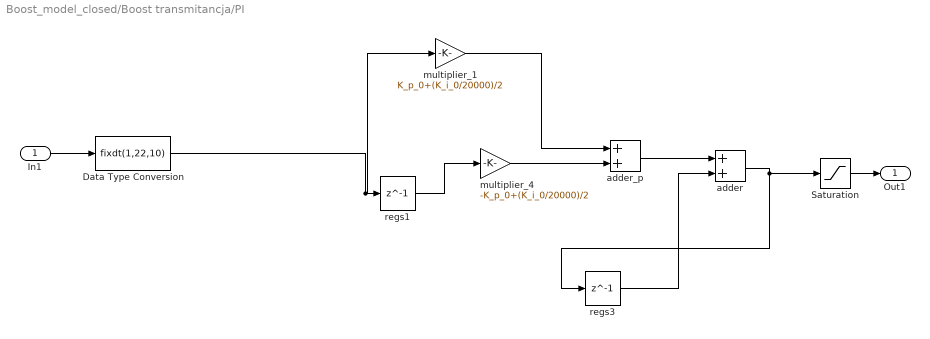
== system Boost_model_closed/Boost transmitancja/PI ==
  In1 : Inport
  Data Type Conversion : DataTypeConversion  OutDataTypeStr=fixdt(1,22,10)
  Saturation : Saturate  UpperLimit=1  LowerLimit=0
  adder : Sum  AccumDataTypeStr=fixdt(1,42,30)  OutDataTypeStr=fixdt(1,42,30)
  adder_p : Sum  AccumDataTypeStr=fixdt(1,42,30)  OutDataTypeStr=fixdt(1,42,30)
  multiplier_1 : Gain  Gain=K_p_0+(K_i_0/20000)/2  ParamDataTypeStr=fixdt(1,21,20)  OutDataTypeStr=fixdt(1,42,30)
  multiplier_4 : Gain  Gain=-K_p_0+(K_i_0/20000)/2  ParamDataTypeStr=fixdt(1,21,20)  OutDataTypeStr=fixdt(1,42,30)
  regs1 : Delay  DelayLength=1  SampleTime=T_PWM
  regs3 : Delay  DelayLength=1  SampleTime=T_PWM
  Out1 : Outport
  wires:
  multiplier_1/1 -> adder_p/1
  multiplier_4/1 -> adder_p/2
  adder/1 -> Saturation/1, regs3/1
  adder_p/1 -> adder/1
  Data Type Conversion/1 -> multiplier_1/1, regs1/1
  regs1/1 -> multiplier_4/1
  regs3/1 -> adder/2
  Saturation/1 -> Out1/1
  In1/1 -> Data Type Conversion/1

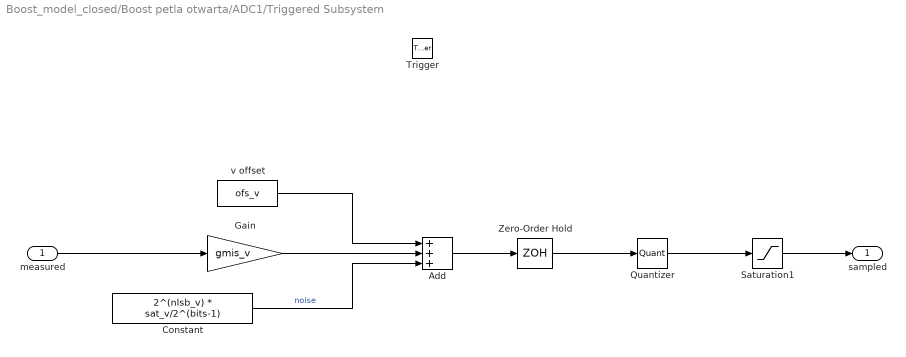
== system Boost_model_closed/Boost petla otwarta/ADC1/Triggered Subsystem ==
  measured : Inport
  Trigger : TriggerPort  VariantControl=Variant
  Add : Sum  Inputs=+++
  Constant : Constant  Value=2^(nlsb_v) * sat_v/2^(bits-1)
  Gain : Gain  Gain=gmis_v
  Quantizer : Quantizer  QuantizationInterval=2* sat_v/2^bits
  Saturation1 : Saturate  UpperLimit=sat_v  LowerLimit=-sat_v
  Zero-Order Hold : ZeroOrderHold  SampleTime=-1
  v offset : Constant  Value=ofs_v
  sampled : Outport  VectorParamsAs1DForOutWhenUnconnected=off
  wires:
  Constant/1 -> Add/3  "noise"
  Saturation1/1 -> sampled/1
  measured/1 -> Gain/1
  Add/1 -> Zero-Order Hold/1
  Gain/1 -> Add/2
  Quantizer/1 -> Saturation1/1
  v offset/1 -> Add/1
  Zero-Order Hold/1 -> Quantizer/1

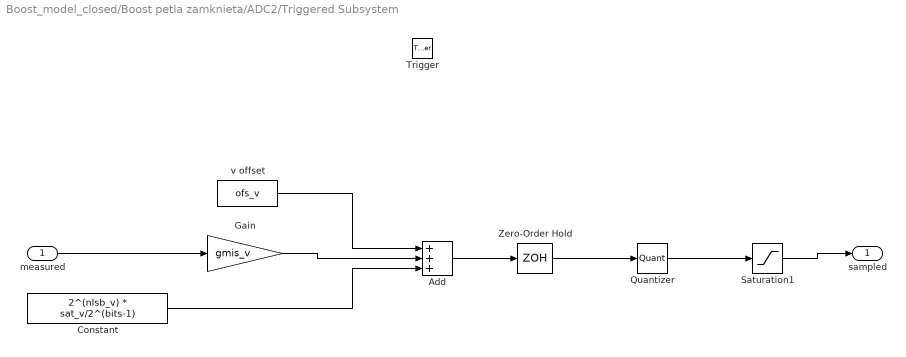
== system Boost_model_closed/Boost petla zamknieta/ADC2/Triggered Subsystem ==
  measured : Inport
  Trigger : TriggerPort  VariantControl=Variant
  Add : Sum  Inputs=+++
  Constant : Constant  Value=2^(nlsb_v) * sat_v/2^(bits-1)
  Gain : Gain  Gain=gmis_v
  Quantizer : Quantizer  QuantizationInterval=2* sat_v/2^bits
  Saturation1 : Saturate  UpperLimit=sat_v  LowerLimit=-sat_v
  Zero-Order Hold : ZeroOrderHold  SampleTime=-1
  v offset : Constant  Value=ofs_v
  sampled : Outport  VectorParamsAs1DForOutWhenUnconnected=off
  wires:
  Saturation1/1 -> sampled/1
  measured/1 -> Gain/1
  Add/1 -> Zero-Order Hold/1
  Gain/1 -> Add/2
  Quantizer/1 -> Saturation1/1
  v offset/1 -> Add/1
  Zero-Order Hold/1 -> Quantizer/1
  Constant/1 -> Add/3
